simulink model "Model_3rdPoint_PID"  (R2023b)
settings: Solver=VariableStepAuto  StartTime=0.0  StopTime=H  RelTol=1e-3
values from neighbouring files (symbols this model uses):
  C_f = c_f*m_f    (= 360000)    [init.m]
  C_f_2 = c_f_2*m_f_2    (= 360000)    [init.m]
  C_f_3 = c_f_3*m_f_3    (= 240000)    [init.m]
  C_f_4 = c_f_4*m_f_4    (= 480000)    [init.m]
  k_fc = barK_fc*s_c    (= 570)    [init.m]
  q_MAX = 20000    [init.m]
  q_MAX_1 = 25000    [init.m]
  q_min = 0    [init.m]
  q_s = barK_fc * a    (= 5.529)    [init.m]
  theta0_f = 280    [init.m]
  Ts = 5    [init.m]
  var_wf = 1    [init.m]
libraries: slpidlib x4
settings Model: Creator=adil2  LastModifiedBy=adil2
settings DataIOCC: ReturnWorkspaceOutputs=off

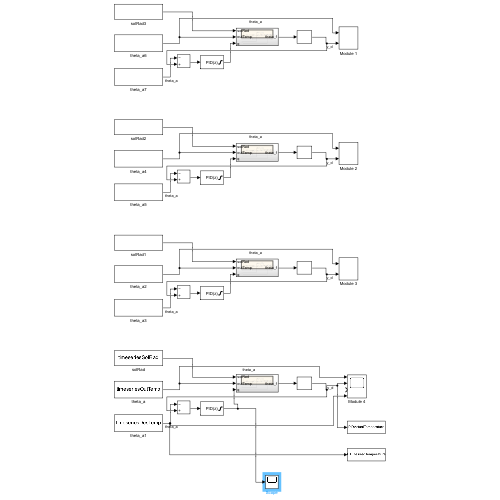
[thumbnail: Simulink's stored preview of the top-level diagram]
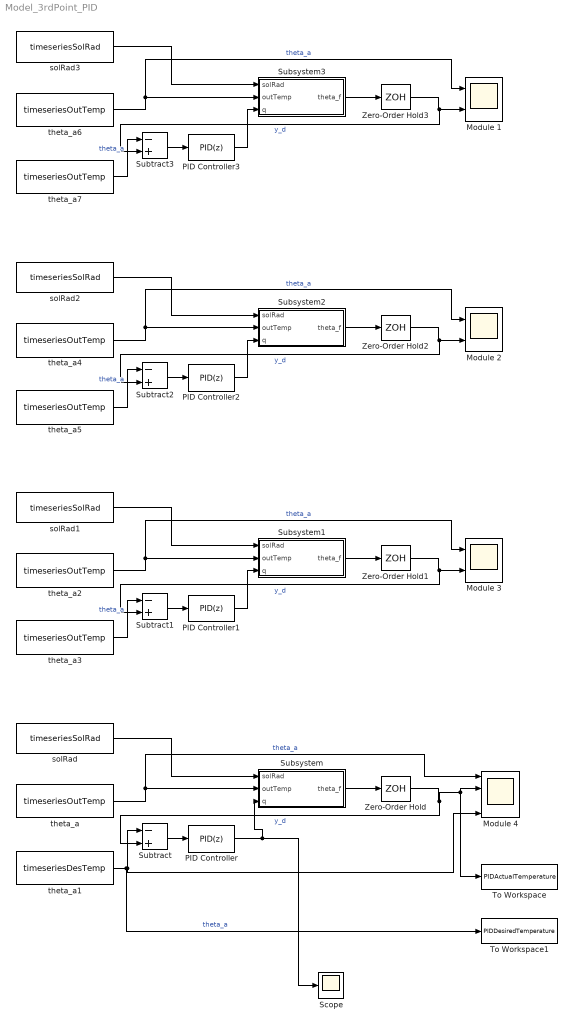
== system Model_3rdPoint_PID ==
  Module 1 : Scope  NumInputPorts=2
  Module 2 : Scope  NumInputPorts=2
  Module 3 : Scope  NumInputPorts=2
  Module 4 : Scope  NumInputPorts=4
  PID Controller : slpidlib/PID Controller  Controller=PID  Form=Parallel  TimeDomain=Discrete-time  UseExternalTs=off  SampleTime=Ts  IntegratorMethod=Forward Euler  FilterMethod=Forward Euler  ControllerParametersSource=internal  P=-769.625340072014  I=-1.82107734947656  UseKiTs=off  D=19125.8641902588  N=0.00360353933336193  UseFilter=on  TunerSelectOption=Transfer Function Based (PID Tuner App)  InitialConditionSource=internal  InitialConditionForIntegrator=0  InitialConditionForFilter=0  DifferentiatorICPrevScaledInput=0  ExternalReset=none  TrackingMode=off  Kt=1  LimitOutput=on  SatLimitsSource=internal  UpperSaturationLimit=q_MAX  LowerSaturationLimit=q_min  LinearizeAsGain=on  AntiWindupMode=none  Kb=1  LimitIntegrator=off  UpperIntegratorSaturationLimit=inf  LowerIntegratorSaturationLimit=-inf  POutMin=[]  POutMax=[]  IOutMin=[]  IOutMax=[]  DOutMin=[]  DOutMax=[]  NOutMin=[]  NOutMax=[]  SumOutMin=[]  SumOutMax=[]  SaturationOutMin=[]  SaturationOutMax=[]  PParamMin=[]  PParamMax=[]  IParamMin=[]  IParamMax=[]  DParamMin=[]  DParamMax=[]  NParamMin=[]  NParamMax=[]  KbParamMin=[]  KbParamMax=[]  KtParamMin=[]  KtParamMax=[]  KbOutMin=[]  KbOutMax=[]  KtOutMin=[]  KtOutMax=[]  IntegratorOutMin=[]  IntegratorOutMax=[]  FilterOutMin=[]  FilterOutMax=[]  SumI1OutMin=[]  SumI1OutMax=[]  SumI2OutMin=[]  SumI2OutMax=[]  SumI3OutMin=[]  SumI3OutMax=[]  SumI4OutMin=[]  SumI4OutMax=[]  SumDOutMin=[]  SumDOutMax=[]  DifferentiatorOutMin=[]  DifferentiatorOutMax=[]  FilterDiffOutCoefMin=[]  FilterDiffOutCoefMax=[]  ReciprocalOutMin=[]  ReciprocalOutMax=[]  SumDenOutMin=[]  SumDenOutMax=[]  SumNumOutMin=[]  SumNumOutMax=[]  DivideOutMin=[]  DivideOutMax=[]  UdiffTsProdOutMin=[]  UdiffTsProdOutMax=[]  NTsProdOutMin=[]  NTsProdOutMax=[]  UintegralTsProdOutMin=[]  UintegralTsProdOutMax=[]  UngainTsProdOutMin=[]  UngainTsProdOutMax=[]  ClampingZeroOutDataTypeStr=Inherit: Inherit via back propagation  ClampingZeroOutMin=[]  ClampingZeroOutMax=[]  FilterDenConstantOutDataTypeStr=Inherit: Inherit via back propagation  FilterDenConstantOutMin=[]  FilterDenConstantOutMax=[]  PCopyOutDataTypeStr=Inherit: Inherit via back propagation  PCopyOutMin=[]  PCopyOutMax=[]  NCopyOutDataTypeStr=Inherit: Inherit via back propagation  NCopyOutMin=[]  NCopyOutMax=[]  IntegratorContinuousStateAttributes=''  IntegratorStateMustResolveToSignalObject=off  IntegratorRTWStateStorageClass=Auto  FilterContinuousStateAttributes=''  FilterStateMustResolveToSignalObject=off  FilterRTWStateStorageClass=Auto  ParallelPVariant=InternalParameters  IdealPVariant=Disabled  IVariant=InternalParameters  DVariant=InternalParameters  IntegratorVariant=Discrete  SatVariant=Enabled  AWVariant=Passthrough  PCopyVariant=Disabled  TRVariant=Disabled  FdbkBlocksVariant=Forward  IdealPFdbkVariant=Disabled  SatFdbkVariant=Disabled  DerivativeFilterVariant=ForwardEulerFilter  NVariant=InternalParameters  NCopyVariant=Disabled  FilterICVariant=InternalICsFilter  IntegratorICVariant=InternalICs  ExternalResetVariant=Disabled  TRSumVariant=Passthrough  SumFdbkVariant=Disabled  SumVariant=Sum_PID  TsampFilterVariant=InternalTs  TsampNgainVariant=Passthrough  TsampIntegralVariant=Disabled_SignalSpec  ExternalSaturationOutDataTypeStr=Inherit: Same as second input
  PID Controller1 : slpidlib/PID Controller  Controller=PID  Form=Parallel  TimeDomain=Discrete-time  UseExternalTs=off  SampleTime=Ts  IntegratorMethod=Forward Euler  FilterMethod=Forward Euler  ControllerParametersSource=internal  P=-834.358128139547  I=-3.78545132097434  UseKiTs=off  D=15793.215424436  N=0.00516191188811559  UseFilter=on  TunerSelectOption=Transfer Function Based (PID Tuner App)  InitialConditionSource=internal  InitialConditionForIntegrator=0  InitialConditionForFilter=0  DifferentiatorICPrevScaledInput=0  ExternalReset=none  TrackingMode=off  Kt=1  LimitOutput=on  SatLimitsSource=internal  UpperSaturationLimit=q_MAX  LowerSaturationLimit=q_min  LinearizeAsGain=on  AntiWindupMode=none  Kb=1  LimitIntegrator=off  UpperIntegratorSaturationLimit=inf  LowerIntegratorSaturationLimit=-inf  POutMin=[]  POutMax=[]  IOutMin=[]  IOutMax=[]  DOutMin=[]  DOutMax=[]  NOutMin=[]  NOutMax=[]  SumOutMin=[]  SumOutMax=[]  SaturationOutMin=[]  SaturationOutMax=[]  PParamMin=[]  PParamMax=[]  IParamMin=[]  IParamMax=[]  DParamMin=[]  DParamMax=[]  NParamMin=[]  NParamMax=[]  KbParamMin=[]  KbParamMax=[]  KtParamMin=[]  KtParamMax=[]  KbOutMin=[]  KbOutMax=[]  KtOutMin=[]  KtOutMax=[]  IntegratorOutMin=[]  IntegratorOutMax=[]  FilterOutMin=[]  FilterOutMax=[]  SumI1OutMin=[]  SumI1OutMax=[]  SumI2OutMin=[]  SumI2OutMax=[]  SumI3OutMin=[]  SumI3OutMax=[]  SumI4OutMin=[]  SumI4OutMax=[]  SumDOutMin=[]  SumDOutMax=[]  DifferentiatorOutMin=[]  DifferentiatorOutMax=[]  FilterDiffOutCoefMin=[]  FilterDiffOutCoefMax=[]  ReciprocalOutMin=[]  ReciprocalOutMax=[]  SumDenOutMin=[]  SumDenOutMax=[]  SumNumOutMin=[]  SumNumOutMax=[]  DivideOutMin=[]  DivideOutMax=[]  UdiffTsProdOutMin=[]  UdiffTsProdOutMax=[]  NTsProdOutMin=[]  NTsProdOutMax=[]  UintegralTsProdOutMin=[]  UintegralTsProdOutMax=[]  UngainTsProdOutMin=[]  UngainTsProdOutMax=[]  ClampingZeroOutDataTypeStr=Inherit: Inherit via back propagation  ClampingZeroOutMin=[]  ClampingZeroOutMax=[]  FilterDenConstantOutDataTypeStr=Inherit: Inherit via back propagation  FilterDenConstantOutMin=[]  FilterDenConstantOutMax=[]  PCopyOutDataTypeStr=Inherit: Inherit via back propagation  PCopyOutMin=[]  PCopyOutMax=[]  NCopyOutDataTypeStr=Inherit: Inherit via back propagation  NCopyOutMin=[]  NCopyOutMax=[]  IntegratorContinuousStateAttributes=''  IntegratorStateMustResolveToSignalObject=off  IntegratorRTWStateStorageClass=Auto  FilterContinuousStateAttributes=''  FilterStateMustResolveToSignalObject=off  FilterRTWStateStorageClass=Auto  ParallelPVariant=InternalParameters  IdealPVariant=Disabled  IVariant=InternalParameters  DVariant=InternalParameters  IntegratorVariant=Discrete  SatVariant=Enabled  AWVariant=Passthrough  PCopyVariant=Disabled  TRVariant=Disabled  FdbkBlocksVariant=Forward  IdealPFdbkVariant=Disabled  SatFdbkVariant=Disabled  DerivativeFilterVariant=ForwardEulerFilter  NVariant=InternalParameters  NCopyVariant=Disabled  FilterICVariant=InternalICsFilter  IntegratorICVariant=InternalICs  ExternalResetVariant=Disabled  TRSumVariant=Passthrough  SumFdbkVariant=Disabled  SumVariant=Sum_PID  TsampFilterVariant=InternalTs  TsampNgainVariant=Passthrough  TsampIntegralVariant=Disabled_SignalSpec  ExternalSaturationOutDataTypeStr=Inherit: Same as second input
  PID Controller2 : slpidlib/PID Controller  Controller=PID  Form=Parallel  TimeDomain=Discrete-time  UseExternalTs=off  SampleTime=Ts  IntegratorMethod=Forward Euler  FilterMethod=Forward Euler  ControllerParametersSource=internal  P=-836.776233915855  I=-2.56232246150505  UseKiTs=off  D=23651.5427743954  N=0.00348551941541599  UseFilter=on  TunerSelectOption=Transfer Function Based (PID Tuner App)  InitialConditionSource=internal  InitialConditionForIntegrator=0  InitialConditionForFilter=0  DifferentiatorICPrevScaledInput=0  ExternalReset=none  TrackingMode=off  Kt=1  LimitOutput=on  SatLimitsSource=internal  UpperSaturationLimit=q_MAX  LowerSaturationLimit=q_min  LinearizeAsGain=on  AntiWindupMode=none  Kb=1  LimitIntegrator=off  UpperIntegratorSaturationLimit=inf  LowerIntegratorSaturationLimit=-inf  POutMin=[]  POutMax=[]  IOutMin=[]  IOutMax=[]  DOutMin=[]  DOutMax=[]  NOutMin=[]  NOutMax=[]  SumOutMin=[]  SumOutMax=[]  SaturationOutMin=[]  SaturationOutMax=[]  PParamMin=[]  PParamMax=[]  IParamMin=[]  IParamMax=[]  DParamMin=[]  DParamMax=[]  NParamMin=[]  NParamMax=[]  KbParamMin=[]  KbParamMax=[]  KtParamMin=[]  KtParamMax=[]  KbOutMin=[]  KbOutMax=[]  KtOutMin=[]  KtOutMax=[]  IntegratorOutMin=[]  IntegratorOutMax=[]  FilterOutMin=[]  FilterOutMax=[]  SumI1OutMin=[]  SumI1OutMax=[]  SumI2OutMin=[]  SumI2OutMax=[]  SumI3OutMin=[]  SumI3OutMax=[]  SumI4OutMin=[]  SumI4OutMax=[]  SumDOutMin=[]  SumDOutMax=[]  DifferentiatorOutMin=[]  DifferentiatorOutMax=[]  FilterDiffOutCoefMin=[]  FilterDiffOutCoefMax=[]  ReciprocalOutMin=[]  ReciprocalOutMax=[]  SumDenOutMin=[]  SumDenOutMax=[]  SumNumOutMin=[]  SumNumOutMax=[]  DivideOutMin=[]  DivideOutMax=[]  UdiffTsProdOutMin=[]  UdiffTsProdOutMax=[]  NTsProdOutMin=[]  NTsProdOutMax=[]  UintegralTsProdOutMin=[]  UintegralTsProdOutMax=[]  UngainTsProdOutMin=[]  UngainTsProdOutMax=[]  ClampingZeroOutDataTypeStr=Inherit: Inherit via back propagation  ClampingZeroOutMin=[]  ClampingZeroOutMax=[]  FilterDenConstantOutDataTypeStr=Inherit: Inherit via back propagation  FilterDenConstantOutMin=[]  FilterDenConstantOutMax=[]  PCopyOutDataTypeStr=Inherit: Inherit via back propagation  PCopyOutMin=[]  PCopyOutMax=[]  NCopyOutDataTypeStr=Inherit: Inherit via back propagation  NCopyOutMin=[]  NCopyOutMax=[]  IntegratorContinuousStateAttributes=''  IntegratorStateMustResolveToSignalObject=off  IntegratorRTWStateStorageClass=Auto  FilterContinuousStateAttributes=''  FilterStateMustResolveToSignalObject=off  FilterRTWStateStorageClass=Auto  ParallelPVariant=InternalParameters  IdealPVariant=Disabled  IVariant=InternalParameters  DVariant=InternalParameters  IntegratorVariant=Discrete  SatVariant=Enabled  AWVariant=Passthrough  PCopyVariant=Disabled  TRVariant=Disabled  FdbkBlocksVariant=Forward  IdealPFdbkVariant=Disabled  SatFdbkVariant=Disabled  DerivativeFilterVariant=ForwardEulerFilter  NVariant=InternalParameters  NCopyVariant=Disabled  FilterICVariant=InternalICsFilter  IntegratorICVariant=InternalICs  ExternalResetVariant=Disabled  TRSumVariant=Passthrough  SumFdbkVariant=Disabled  SumVariant=Sum_PID  TsampFilterVariant=InternalTs  TsampNgainVariant=Passthrough  TsampIntegralVariant=Disabled_SignalSpec  ExternalSaturationOutDataTypeStr=Inherit: Same as second input
  PID Controller3 : slpidlib/PID Controller  Controller=PID  Form=Parallel  TimeDomain=Discrete-time  UseExternalTs=off  SampleTime=Ts  IntegratorMethod=Forward Euler  FilterMethod=Forward Euler  ControllerParametersSource=internal  P=-836.776233915855  I=-2.56232246150505  UseKiTs=off  D=23651.5427743954  N=0.00348551941541599  UseFilter=on  TunerSelectOption=Transfer Function Based (PID Tuner App)  InitialConditionSource=internal  InitialConditionForIntegrator=0  InitialConditionForFilter=0  DifferentiatorICPrevScaledInput=0  ExternalReset=none  TrackingMode=off  Kt=1  LimitOutput=on  SatLimitsSource=internal  UpperSaturationLimit=q_MAX_1  LowerSaturationLimit=q_min  LinearizeAsGain=on  AntiWindupMode=none  Kb=1  LimitIntegrator=off  UpperIntegratorSaturationLimit=inf  LowerIntegratorSaturationLimit=-inf  POutMin=[]  POutMax=[]  IOutMin=[]  IOutMax=[]  DOutMin=[]  DOutMax=[]  NOutMin=[]  NOutMax=[]  SumOutMin=[]  SumOutMax=[]  SaturationOutMin=[]  SaturationOutMax=[]  PParamMin=[]  PParamMax=[]  IParamMin=[]  IParamMax=[]  DParamMin=[]  DParamMax=[]  NParamMin=[]  NParamMax=[]  KbParamMin=[]  KbParamMax=[]  KtParamMin=[]  KtParamMax=[]  KbOutMin=[]  KbOutMax=[]  KtOutMin=[]  KtOutMax=[]  IntegratorOutMin=[]  IntegratorOutMax=[]  FilterOutMin=[]  FilterOutMax=[]  SumI1OutMin=[]  SumI1OutMax=[]  SumI2OutMin=[]  SumI2OutMax=[]  SumI3OutMin=[]  SumI3OutMax=[]  SumI4OutMin=[]  SumI4OutMax=[]  SumDOutMin=[]  SumDOutMax=[]  DifferentiatorOutMin=[]  DifferentiatorOutMax=[]  FilterDiffOutCoefMin=[]  FilterDiffOutCoefMax=[]  ReciprocalOutMin=[]  ReciprocalOutMax=[]  SumDenOutMin=[]  SumDenOutMax=[]  SumNumOutMin=[]  SumNumOutMax=[]  DivideOutMin=[]  DivideOutMax=[]  UdiffTsProdOutMin=[]  UdiffTsProdOutMax=[]  NTsProdOutMin=[]  NTsProdOutMax=[]  UintegralTsProdOutMin=[]  UintegralTsProdOutMax=[]  UngainTsProdOutMin=[]  UngainTsProdOutMax=[]  ClampingZeroOutDataTypeStr=Inherit: Inherit via back propagation  ClampingZeroOutMin=[]  ClampingZeroOutMax=[]  FilterDenConstantOutDataTypeStr=Inherit: Inherit via back propagation  FilterDenConstantOutMin=[]  FilterDenConstantOutMax=[]  PCopyOutDataTypeStr=Inherit: Inherit via back propagation  PCopyOutMin=[]  PCopyOutMax=[]  NCopyOutDataTypeStr=Inherit: Inherit via back propagation  NCopyOutMin=[]  NCopyOutMax=[]  IntegratorContinuousStateAttributes=''  IntegratorStateMustResolveToSignalObject=off  IntegratorRTWStateStorageClass=Auto  FilterContinuousStateAttributes=''  FilterStateMustResolveToSignalObject=off  FilterRTWStateStorageClass=Auto  ParallelPVariant=InternalParameters  IdealPVariant=Disabled  IVariant=InternalParameters  DVariant=InternalParameters  IntegratorVariant=Discrete  SatVariant=Enabled  AWVariant=Passthrough  PCopyVariant=Disabled  TRVariant=Disabled  FdbkBlocksVariant=Forward  IdealPFdbkVariant=Disabled  SatFdbkVariant=Disabled  DerivativeFilterVariant=ForwardEulerFilter  NVariant=InternalParameters  NCopyVariant=Disabled  FilterICVariant=InternalICsFilter  IntegratorICVariant=InternalICs  ExternalResetVariant=Disabled  TRSumVariant=Passthrough  SumFdbkVariant=Disabled  SumVariant=Sum_PID  TsampFilterVariant=InternalTs  TsampNgainVariant=Passthrough  TsampIntegralVariant=Disabled_SignalSpec  ExternalSaturationOutDataTypeStr=Inherit: Same as second input
  Scope : Scope
  Subsystem : Subsystem
  Subsystem1 : Subsystem
  Subsystem2 : Subsystem
  Subsystem3 : Subsystem
  Subtract{,1..3} (4 alike) : Sum  Inputs=-+
  To Workspace : ToWorkspace  VariableName=PIDActualTemperature  SampleTime=-1
  To Workspace1 : ToWorkspace  VariableName=PIDDesiredTemperature  SampleTime=-1
  Zero-Order Hold{,1..3} (4 alike) : ZeroOrderHold  SampleTime=Ts
  solRad{,1..3} (4 alike) : FromWorkspace  VariableName=timeseriesSolRad
  theta_a{,2..7} (7 alike) : FromWorkspace  VariableName=timeseriesOutTemp  SampleTime=Ts
  theta_a1 : FromWorkspace  VariableName=timeseriesDesTemp  SampleTime=Ts
  wires:
  Subsystem/1(theta_f) -> Zero-Order Hold/1
  Zero-Order Hold/1 -> Subtract/2, To Workspace/1, Module 4/2  "y_d"
  solRad/1 -> Subsystem/1(solRad)
  theta_a/1 -> Subsystem/2(outTemp), Module 4/1  "theta_a"
  theta_a1/1 -> To Workspace1/1, Subtract/1, Module 4/4  "theta_a"
  Subtract/1 -> PID Controller/1
  PID Controller/1 -> Scope/1, Subsystem/3(q)
  theta_a3/1 -> Subtract1/1  "theta_a"
  Subtract1/1 -> PID Controller1/1
  PID Controller1/1 -> Subsystem1/3(q)
  Zero-Order Hold1/1 -> Subtract1/2, Module 3/2  "y_d"
  theta_a2/1 -> Subsystem1/2(outTemp), Module 3/1  "theta_a"
  Subsystem1/1(theta_f) -> Zero-Order Hold1/1
  solRad1/1 -> Subsystem1/1(solRad)
  solRad2/1 -> Subsystem2/1(solRad)
  PID Controller2/1 -> Subsystem2/3(q)
  Zero-Order Hold2/1 -> Subtract2/2, Module 2/2  "y_d"
  Subsystem2/1(theta_f) -> Zero-Order Hold2/1
  Subtract2/1 -> PID Controller2/1
  theta_a4/1 -> Subsystem2/2(outTemp), Module 2/1  "theta_a"
  theta_a5/1 -> Subtract2/1  "theta_a"
  Zero-Order Hold3/1 -> Subtract3/2, Module 1/2  "y_d"
  theta_a6/1 -> Subsystem3/2(outTemp), Module 1/1  "theta_a"
  theta_a7/1 -> Subtract3/1  "theta_a"
  Subsystem3/1(theta_f) -> Zero-Order Hold3/1
  PID Controller3/1 -> Subsystem3/3(q)
  solRad3/1 -> Subsystem3/1(solRad)
  Subtract3/1 -> PID Controller3/1

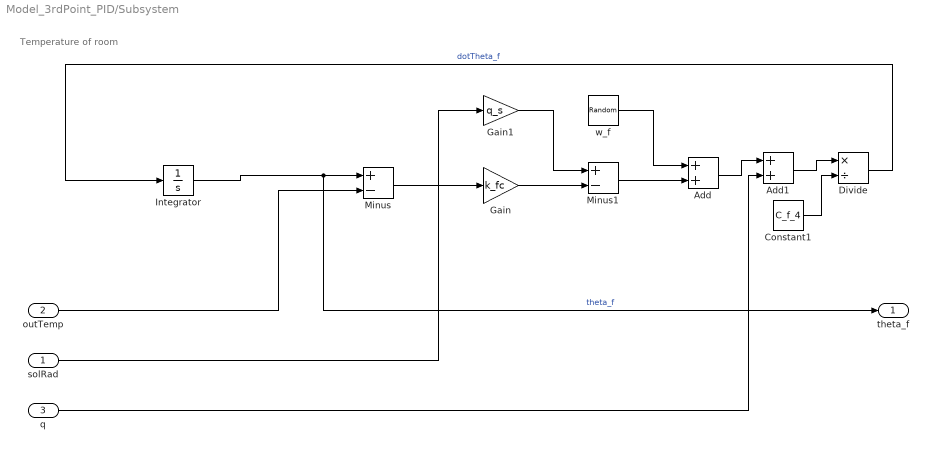
== system Model_3rdPoint_PID/Subsystem ==
  note: Temperature of room
  solRad : Inport
  outTemp : Inport  Port=2
  q : Inport  Port=3
  Add : Sum
  Add1 : Sum
  Constant1 : Constant  Value=C_f_4
  Divide : Product  Inputs=*/
  Gain : Gain  Gain=k_fc
  Gain1 : Gain  Gain=q_s
  Integrator : Integrator  InitialCondition=theta0_f
  Minus : Sum  Inputs=+-
  Minus1 : Sum  Inputs=+-
  w_f : RandomNumber  Variance=var_wf  SampleTime=Ts
  theta_f : Outport
  wires:
  outTemp/1 -> Minus/2
  Integrator/1 -> theta_f/1, Minus/1  "theta_f"
  Minus/1 -> Gain/1
  Constant1/1 -> Divide/2
  Divide/1 -> Integrator/1  "dotTheta_f"
  Gain/1 -> Minus1/2
  Minus1/1 -> Add/2
  w_f/1 -> Add/1
  solRad/1 -> Gain1/1
  Gain1/1 -> Minus1/1
  Add1/1 -> Divide/1
  Add/1 -> Add1/1
  q/1 -> Add1/2

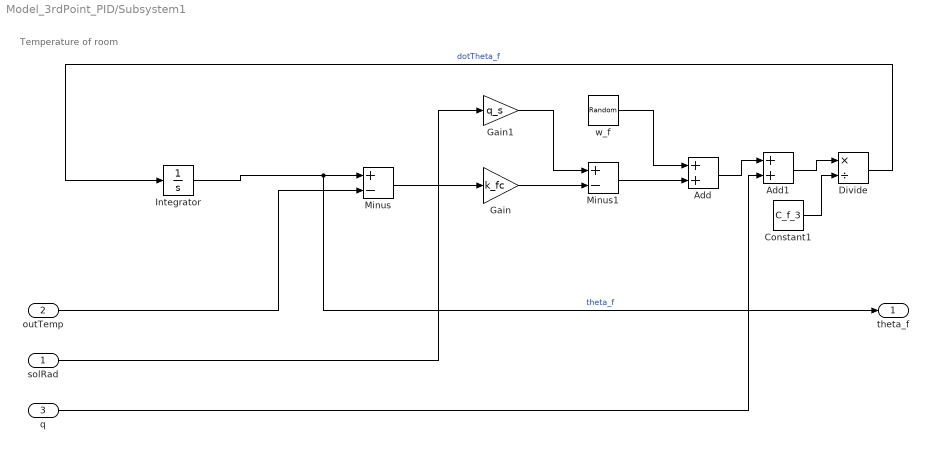
== system Model_3rdPoint_PID/Subsystem1 ==
  note: Temperature of room
  solRad : Inport
  outTemp : Inport  Port=2
  q : Inport  Port=3
  Add : Sum
  Add1 : Sum
  Constant1 : Constant  Value=C_f_3
  Divide : Product  Inputs=*/
  Gain : Gain  Gain=k_fc
  Gain1 : Gain  Gain=q_s
  Integrator : Integrator  InitialCondition=theta0_f
  Minus : Sum  Inputs=+-
  Minus1 : Sum  Inputs=+-
  w_f : RandomNumber  Variance=var_wf  SampleTime=Ts
  theta_f : Outport
  wires:
  outTemp/1 -> Minus/2
  Integrator/1 -> theta_f/1, Minus/1  "theta_f"
  Minus/1 -> Gain/1
  Constant1/1 -> Divide/2
  Divide/1 -> Integrator/1  "dotTheta_f"
  Gain/1 -> Minus1/2
  Minus1/1 -> Add/2
  w_f/1 -> Add/1
  solRad/1 -> Gain1/1
  Gain1/1 -> Minus1/1
  Add1/1 -> Divide/1
  Add/1 -> Add1/1
  q/1 -> Add1/2

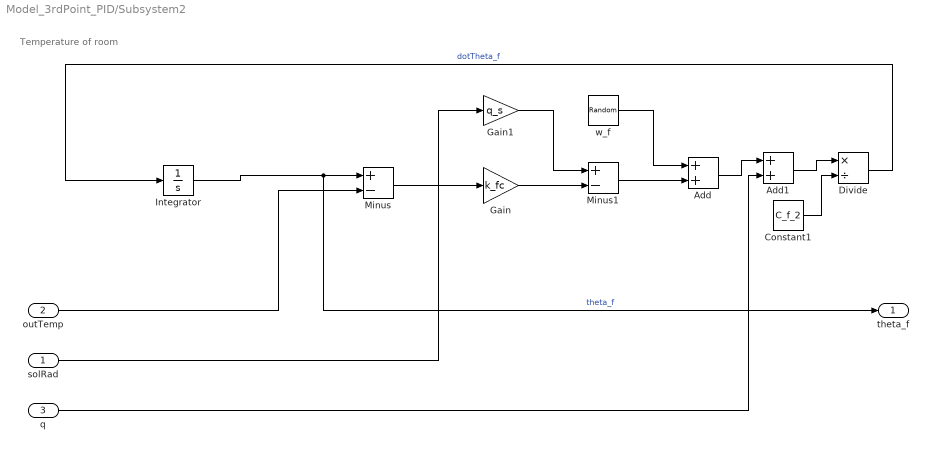
== system Model_3rdPoint_PID/Subsystem2 ==
  note: Temperature of room
  solRad : Inport
  outTemp : Inport  Port=2
  q : Inport  Port=3
  Add : Sum
  Add1 : Sum
  Constant1 : Constant  Value=C_f_2
  Divide : Product  Inputs=*/
  Gain : Gain  Gain=k_fc
  Gain1 : Gain  Gain=q_s
  Integrator : Integrator  InitialCondition=theta0_f
  Minus : Sum  Inputs=+-
  Minus1 : Sum  Inputs=+-
  w_f : RandomNumber  Variance=var_wf  SampleTime=Ts
  theta_f : Outport
  wires:
  outTemp/1 -> Minus/2
  Integrator/1 -> theta_f/1, Minus/1  "theta_f"
  Minus/1 -> Gain/1
  Constant1/1 -> Divide/2
  Divide/1 -> Integrator/1  "dotTheta_f"
  Gain/1 -> Minus1/2
  Minus1/1 -> Add/2
  w_f/1 -> Add/1
  solRad/1 -> Gain1/1
  Gain1/1 -> Minus1/1
  Add1/1 -> Divide/1
  Add/1 -> Add1/1
  q/1 -> Add1/2

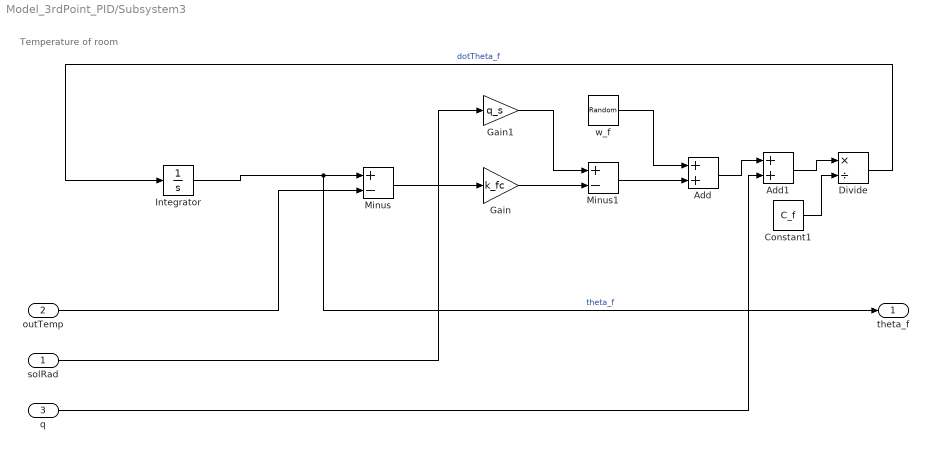
== system Model_3rdPoint_PID/Subsystem3 ==
  note: Temperature of room
  solRad : Inport
  outTemp : Inport  Port=2
  q : Inport  Port=3
  Add : Sum
  Add1 : Sum
  Constant1 : Constant  Value=C_f
  Divide : Product  Inputs=*/
  Gain : Gain  Gain=k_fc
  Gain1 : Gain  Gain=q_s
  Integrator : Integrator  InitialCondition=theta0_f
  Minus : Sum  Inputs=+-
  Minus1 : Sum  Inputs=+-
  w_f : RandomNumber  Variance=var_wf  SampleTime=Ts
  theta_f : Outport
  wires:
  outTemp/1 -> Minus/2
  Integrator/1 -> theta_f/1, Minus/1  "theta_f"
  Minus/1 -> Gain/1
  Constant1/1 -> Divide/2
  Divide/1 -> Integrator/1  "dotTheta_f"
  Gain/1 -> Minus1/2
  Minus1/1 -> Add/2
  w_f/1 -> Add/1
  solRad/1 -> Gain1/1
  Gain1/1 -> Minus1/1
  Add1/1 -> Divide/1
  Add/1 -> Add1/1
  q/1 -> Add1/2
